simulink model "lab5s"  (R2024b)
settings: Solver=VariableStepAuto  StartTime=0.0  StopTime=10.0  MaxStep=0.01  RelTol=1e-3
values from neighbouring files (symbols this model uses):
  x = tab_x(i)    [lab5.m]
  x_prim = tab_dx(i)    [lab5.m]
settings Model: Creator=Adam  LastModifiedBy=Adam

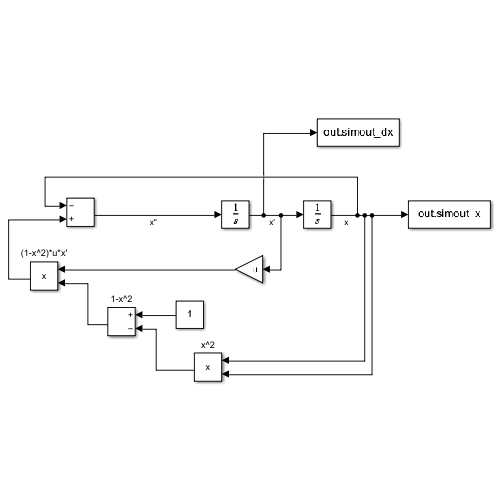
[thumbnail: Simulink's stored preview of the top-level diagram]
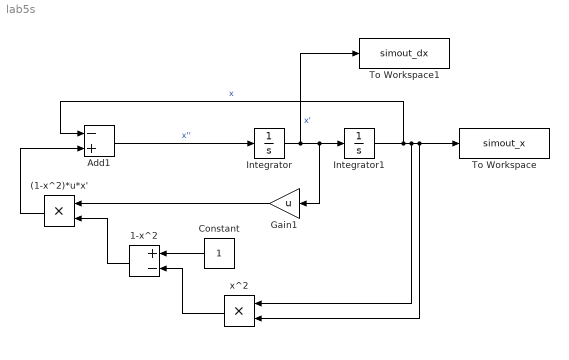
== system lab5s ==
  (1-x^2)*u*x' : Product
  1-x^2 : Sum  Inputs=+-
  Add1 : Sum  Inputs=-+
  Constant : Constant
  Gain1 : Gain  Gain=u
  Integrator : Integrator  InitialCondition=x_prim
  Integrator1 : Integrator  InitialCondition=x
  To Workspace : ToWorkspace  VariableName=simout_x  SampleTime=-1
  To Workspace1 : ToWorkspace  VariableName=simout_dx  SampleTime=-1
  x^2 : Product
  wires:
  Integrator/1 -> To Workspace1/1, Gain1/1, Integrator1/1  "x'"
  Integrator1/1 -> Add1/1, x^2/1, x^2/2, To Workspace/1  "x"
  Constant/1 -> 1-x^2/1
  x^2/1 -> 1-x^2/2
  1-x^2/1 -> (1-x^2)*u*x'/2
  (1-x^2)*u*x'/1 -> Add1/2
  Add1/1 -> Integrator/1  "x''"
  Gain1/1 -> (1-x^2)*u*x'/1
